simulink library "sm_excv_underc_lib"  (R2023b)
settings: Solver=VariableStepAuto  StartTime=0.0  StopTime=10.0  RelTol=1e-3
undefined symbols (not defined in the file): Excv, L1, L2, L3, L4, L5, L6, L7, L8, L9, P1, P2, P3, P4, P5, P6, P7, P8, P9, shoe_w, X, Y, Z
libraries: sm_tracked_vehicle_lib x70, sm_lib x54, nesl_utility x32, sm_excv_scene_lib x9, fl_lib x8, sm_excv_frame_lib x4
(part 1 of 5)
Description:
  | Copyright 2023 The MathWorks, Inc.
settings Model: Creator=smiller  LastModifiedBy=smiller

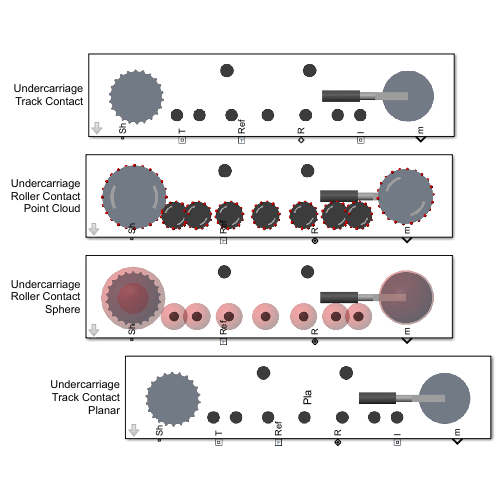
[thumbnail: Simulink's stored preview of the top-level diagram]
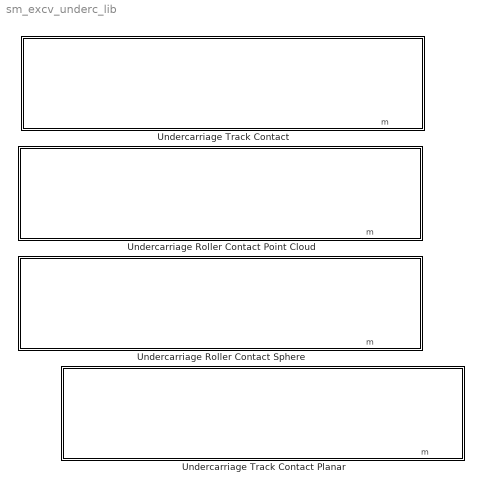
== system sm_excv_underc_lib ==
  Undercarriage Roller Contact Point Cloud : Subsystem  mask(Undercarriage with Roller Ground Contact (Point Cloud)){sprk_xc=Excv.Sprocket.sprocket_xc, sprk_len=Excv.Sprocket.sprk_width, sprk_rho=Excv.Sprocket.density, sprk_clr=Excv.Sprocket.clr, sprk_opc=Excv.Sprocket.opc, sprk_contact_geo_ptcld=Excv.Sprocket.ground_contact.ptcld.pts, sprk_contact_geo_rad=Excv.Sprocket.ground_contact.ptcld.rad, sprk_contact_geo_clr=Excv.Sprocket.ground_contact.ptcld.clr, sprk_contact_geo_opc=Excv.Sprocket.ground_contact.ptcld.opc, idler_rad=Excv.Idler.rad, idler_len=Excv.Idler.len, idler_rho=Excv.Idler.rho, idler_clr=Excv.Idler.clr, idler_opc=Excv.Idler.opc, idler_contact_geo_ptcld=Excv.Idler.ground_contact.ptcld.pts, idler_contact_geo_rad=Excv.Idler.ground_contact.ptcld.rad, idler_contact_geo_clr=Excv.Idler.ground_contact.ptcld.clr, idler_contact_geo_opc=Excv.Idler.ground_contact.ptcld.opc, roller_upper_rad=Excv.Roller.Upper.rad, roller_upper_len=Excv.Roller.Upper.len, roller_upper_rho=Excv.Roller.Upper.rho, roller_upper_clr=Excv.Roller.Upper.clr, roller_upper_opc=Excv.Roller.Upper.opc, roller_upper_contgeo_clr=[1.0 0.0 0.0], roller_upper_contgeo_opc=1, roller_lower_rad=Excv.Roller.Lower.rad, roller_lower_len=Excv.Roller.Lower.len, roller_lower_rho=Excv.Roller.Lower.rho, roller_lower_clr=Excv.Roller.Lower.clr, roller_lower_opc=Excv.Roller.Lower.opc, roller_lower_contgeo_ptcld=Excv.Roller.Lower.ground_contact.ptcld.pts, roller_lower_contgeo_rad=Excv.Roller.Lower.ground_contact.ptcld.rad, roller_lower_contgeo_clr=Excv.Roller.Lower.ground_contact.ptcld.clr, roller_lower_contgeo_opc=Excv.Roller.Lower.ground_contact.ptcld.opc, tensioner_cyl_len=Excv.Idler.Tensioner.cyl.len, tensioner_cyl_rad=Excv.Idler.Tensioner.cyl.rad, tensioner_cyl_rho=Excv.Idler.Tensioner.cyl.rho, tensioner_cyl_clr=Excv.Idler.Tensioner.cyl.clr, tensioner_cyl_opc=Excv.Idler.Tensioner.cyl.opc, tensioner_pist_len=Excv.Idler.Tensioner.piston.len, tensioner_pist_rad=Excv.Idler.Tensioner.piston.rad, tensioner_pist_rho=Excv.Idler.Tensioner.piston.rho, tensioner_pist_clr=Excv.Idler.Tensioner.piston.clr, tensioner_pist_opc=Excv.Idler.Tensioner.piston.opc, tensioner_br_length=Excv.Idler.Tensioner.bracket.len, tensioner_br_width=Excv.Idler.Tensioner.bracket.wid, tensioner_br_height=Excv.Idler.Tensioner.bracket.height, tensioner_br_thk=Excv.Idler.Tensioner.bracket.thk, tensioner_br_rho=Excv.Idler.Tensioner.bracket.rho, tensioner_br_clr=Excv.Idler.Tensioner.bracket.clr, tensioner_br_opc=Excv.Idler.Tensioner.bracket.opc, idler_max_ext=Excv.Idler.Tensioner.cyl.max_ext, sprk_rolling_rad=Excv.Sprocket.ground_contact.rolling_radius, idler_rolling_rad=Excv.Idler.ground_contact.rolling_radius, roller_lower_rolling_rad=Excv.Roller.Lower.ground_contact.rolling_radius, cyl_len=Excv.Shoe.w, lext=1e-3, roller_cyl_clr=Excv.Roller.Lower.clr, roller_cyl_opc=1, sprocket_cyl_clr=Excv.Sprocket.clr, sprocket_cyl_opc=1, idler_cyl_clr=Excv.Idler.clr, idler_cyl_opc=1, accMn=0.65, accMx=0.75, acc_clr=[0.8 0.8 0.8], acc_opc=1, roller_upper_x=Excv.Frame.Sprk2UpperX, roller_lower_x=Excv.Frame.Sprk2LowerX, idler_x=Excv.Frame.IdlerAssyX, roller_upper_y=Excv.Frame.Sprk2UpperY, plate_h=Excv.Chain.plate_h, sprk_pitch_rad=Excv.Sprocket.sprocket_rPitch, idler_lower_roller_offset_y=Excv.Frame.IdlerRollerVoffset, popup_sense_roller=Actuator Torque}
      mask prompts: sprk_xc "Extrusion Data [x y] (m)"; sprk_len "Length (m)"; sprk_rho "Density (kg/m^3)"; sprk_clr "Color [R G B] (0-1)"; sprk_opc "Opacity (0-1)"; sprk_contact_geo_ptcld "Point Cloud Data [x y z] (m)"; sprk_contact_geo_rad "Radius (m)"; sprk_contact_geo_clr "Color [R G B] (0-1)"; sprk_contact_geo_opc "Opacity (0-1)"; idler_rad "Idler Radius (m)"; idler_len "Length (m)"; idler_rho "Density (kg/m^3)"; idler_clr "Color [R G B] (0-1)"; idler_opc "Opacity (0-1)"; idler_contact_geo_ptcld "Point Cloud Data [x y z] (m)"; idler_contact_geo_rad "Point Radius (m)"; idler_contact_geo_clr "Color [R G B] (0-1)"; idler_contact_geo_opc "Opacity (0-1)"; roller_upper_rad "Radius (m)"; roller_upper_len "Length (m)"; roller_upper_rho "Density (kg/m^3)"; roller_upper_clr "Color [R G B] (0-1)"; roller_upper_opc "Opacity (0-1)"; roller_upper_contgeo_clr "Color [R G B] (0-1)"; roller_upper_contgeo_opc "Opacity (0-1)"; roller_lower_rad "Lower Roller Radius (m)"; roller_lower_len "Length (m)"; roller_lower_rho "Density (kg/m^3)"; roller_lower_clr "Color [R G B] (0-1)"; roller_lower_opc "Opacity (0-1)"; roller_lower_contgeo_ptcld "Point Cloud [x y z] (m)"; roller_lower_contgeo_rad "Point Radius (m)"; roller_lower_contgeo_clr "Color [R G B] (0-1)"; roller_lower_contgeo_opc "Opacity (0-1)"; tensioner_cyl_len "Length (m)"; tensioner_cyl_rad "Radius (m)"; tensioner_cyl_rho "Density (kg/m^3)"; tensioner_cyl_clr "Color [R G B] (0-1)"; tensioner_cyl_opc "Opacity (0-1)"; tensioner_pist_len "Length (m)"; tensioner_pist_rad "Radius (m)"; tensioner_pist_rho "Density (kg/m^3)"; tensioner_pist_clr "Color [R G B] (0-1)"; tensioner_pist_opc "Opacity (0.1)"; tensioner_br_length "Length (m)"; tensioner_br_width "Width (m)"; tensioner_br_height "Height (m)"; tensioner_br_thk "Thickness (m)"; tensioner_br_rho "Density (kg/m^3)"; tensioner_br_clr "Color [R G B] (0-1)"; tensioner_br_opc "Opacity (0.1)"; idler_max_ext "Max Extension in Track (m)"; sprk_rolling_rad "Sprocket Rolling Radius (m)"; idler_rolling_rad "Idler Rolling Radius (m)"; roller_lower_rolling_rad "Lower Roller Rolling Radius (m)"; cyl_len "Track Width (m)"; lext "Length Extensions (m)"; roller_cyl_clr "Cylinder Color [R G B] (0-1)"; roller_cyl_opc "Cylinder Opacity (0-1)"; sprocket_cyl_clr "Cylinder Color [R G B] (0-1)"; sprocket_cyl_opc "Cylinder Opacity (0-1)"; idler_cyl_clr "Cylinder Color [R G B] (0-1)"; idler_cyl_opc "Cylinder Opacity (0-1)"; accMn "Accent Min Radius (0-1)"; accMx "Accent Max Radius (0-1)"; acc_clr "Accent Color [R G B] (0-1)"; acc_opc "Accent Opacity (0-1)"; roller_upper_x "Upper Rollers (vector) (m)"; roller_lower_x "Lower Rollers (vector) (m)"; idler_x "Idler Wheel (m)"; roller_upper_y "Sprocket to Upper Rollers (m)"; plate_h "Chain Plate Height (m)"; sprk_pitch_rad "Sprocket Pitch Radius (m)"; idler_lower_roller_offset_y "Idler to Lower Roller Offset (lower edge) (m)"; popup_sense_roller "Roller"
      mask help: Models sprocket, rollers, and idler. Components have point cloud contact geometry to enable undercarriage to roll along uneven ground. The sprocket has a 1D rotational mechanical interface to the drivetrain.
      mask TypeOptions sprk_xc: Rollers/sprk_xc
      mask TypeOptions sprk_len: Rollers/sprk_len
      mask TypeOptions sprk_rho: Rollers/sprk_rho
      mask TypeOptions sprk_clr: Rollers/sprk_clr
      mask TypeOptions sprk_opc: Rollers/sprk_opc
      mask TypeOptions sprk_contact_geo_ptcld: Rollers/sprk_contact_geo_ptcld
      mask TypeOptions sprk_contact_geo_rad: Rollers/sprk_contact_geo_rad
      mask TypeOptions sprk_contact_geo_clr: Rollers/sprk_contact_geo_clr
      mask TypeOptions sprk_contact_geo_opc: Rollers/sprk_contact_geo_opc
      mask TypeOptions idler_rad: Frame/idler_rad | Rollers/idler_rad
      mask TypeOptions idler_len: Rollers/idler_len
      mask TypeOptions idler_rho: Rollers/idler_rho
      mask TypeOptions idler_clr: Rollers/idler_clr
      mask TypeOptions idler_opc: Rollers/idler_opc
      mask TypeOptions idler_contact_geo_ptcld: Rollers/idler_contact_geo_ptcld
      mask TypeOptions idler_contact_geo_rad: Rollers/idler_contact_geo_rad
      mask TypeOptions idler_contact_geo_clr: Rollers/idler_contact_geo_clr
      mask TypeOptions idler_contact_geo_opc: Rollers/idler_contact_geo_opc
      mask TypeOptions roller_upper_rad: Rollers/roller_upper_rad
      mask TypeOptions roller_upper_len: Rollers/roller_upper_len
      mask TypeOptions roller_upper_rho: Rollers/roller_upper_rho
      mask TypeOptions roller_upper_clr: Rollers/roller_upper_clr
      mask TypeOptions roller_upper_opc: Rollers/roller_upper_opc
      mask TypeOptions roller_upper_contgeo_clr: Rollers/roller_upper_contgeo_clr
      mask TypeOptions roller_upper_contgeo_opc: Rollers/roller_upper_contgeo_opc
      mask TypeOptions roller_lower_rad: Frame/roller_lower_rad | Rollers/roller_lower_rad
      mask TypeOptions roller_lower_len: Rollers/roller_lower_len
      mask TypeOptions roller_lower_rho: Rollers/roller_lower_rho
      mask TypeOptions roller_lower_clr: Rollers/roller_lower_clr
      mask TypeOptions roller_lower_opc: Rollers/roller_lower_opc
      mask TypeOptions roller_lower_contgeo_ptcld: Rollers/roller_lower_contgeo_ptcld
      mask TypeOptions roller_lower_contgeo_rad: Rollers/roller_lower_contgeo_rad
      mask TypeOptions roller_lower_contgeo_clr: Rollers/roller_lower_contgeo_clr
      mask TypeOptions roller_lower_contgeo_opc: Rollers/roller_lower_contgeo_opc
      mask TypeOptions tensioner_cyl_len: Rollers/tensioner_cyl_len
      mask TypeOptions tensioner_cyl_rad: Rollers/tensioner_cyl_rad
      mask TypeOptions tensioner_cyl_rho: Rollers/tensioner_cyl_rho
      mask TypeOptions tensioner_cyl_clr: Rollers/tensioner_cyl_clr
      mask TypeOptions tensioner_cyl_opc: Rollers/tensioner_cyl_opc
      mask TypeOptions tensioner_pist_len: Rollers/tensioner_pist_len
      mask TypeOptions tensioner_pist_rad: Rollers/tensioner_pist_rad
      mask TypeOptions tensioner_pist_rho: Rollers/tensioner_pist_rho
      mask TypeOptions tensioner_pist_clr: Rollers/tensioner_pist_clr
      mask TypeOptions tensioner_pist_opc: Rollers/tensioner_pist_opc
      mask TypeOptions tensioner_br_length: Rollers/tensioner_br_length
      mask TypeOptions tensioner_br_width: Rollers/tensioner_br_width
      mask TypeOptions tensioner_br_height: Rollers/tensioner_br_height
      mask TypeOptions tensioner_br_thk: Rollers/tensioner_br_thk
      mask TypeOptions tensioner_br_rho: Rollers/tensioner_br_rho
      mask TypeOptions tensioner_br_clr: Rollers/tensioner_br_clr
      mask TypeOptions tensioner_br_opc: Rollers/tensioner_br_opc
      mask TypeOptions idler_max_ext: Rollers/idler_max_ext
      mask TypeOptions sprk_rolling_rad: Rollers/sprk_rolling_rad
      mask TypeOptions idler_rolling_rad: Rollers/idler_rolling_rad
      mask TypeOptions roller_lower_rolling_rad: Rollers/roller_lower_rolling_rad
      mask TypeOptions cyl_len: Rollers/cyl_len
      mask TypeOptions lext: Rollers/lext
      mask TypeOptions roller_cyl_clr: Rollers/roller_cyl_clr
      mask TypeOptions roller_cyl_opc: Rollers/roller_cyl_opc
      mask TypeOptions sprocket_cyl_clr: Rollers/sprocket_cyl_clr
      mask TypeOptions sprocket_cyl_opc: Rollers/sprocket_cyl_opc
      mask TypeOptions idler_cyl_clr: Rollers/idler_cyl_clr
      mask TypeOptions idler_cyl_opc: Rollers/idler_cyl_opc
      mask TypeOptions accMn: Rollers/accMn
      mask TypeOptions accMx: Rollers/accMx
      mask TypeOptions acc_clr: Rollers/acc_clr
      mask TypeOptions acc_opc: Rollers/acc_opc
      mask TypeOptions roller_upper_x: Frame/roller_upper_x
      mask TypeOptions roller_lower_x: Frame/roller_lower_x
      mask TypeOptions idler_x: Frame/idler_x
      mask TypeOptions roller_upper_y: Frame/roller_upper_y
      mask TypeOptions plate_h: Frame/plate_h
      mask TypeOptions sprk_pitch_rad: Frame/sprk_pitch_rad
      mask TypeOptions idler_lower_roller_offset_y: Frame/idler_lower_roller_offset_y
      mask TypeOptions popup_sense_roller: Rollers/popup_sense_roller
      mask DialogControl cont_sprocket Prompt: Sprocket
      mask DialogControl cont_sprocket_solid Prompt: Solid
      mask DialogControl cont_sprocket_contact_geo Prompt: Contact Geometry
      mask DialogControl cont_idler Prompt: Idler
      mask DialogControl cont_idler_solid Prompt: Solid
      mask DialogControl cont_idler_contact_geo Prompt: Contact Geometry
      mask DialogControl cont_rollers Prompt: Rollers
      mask DialogControl cont_roller_upper Prompt: Upper
      mask DialogControl cont_roller_upper_contact_geo Prompt: Contact Geometry
      mask DialogControl cont_rollers_lower Prompt: Lower
      mask DialogControl cont_rollers_lower_contact_geo Prompt: Contact Geometry
      mask DialogControl cont_tensioner Prompt: Tensioner
      mask DialogControl cont_tensioner_cyl Prompt: Cylinder
      mask DialogControl cont_tensioner_pist Prompt: Piston
      mask DialogControl cont_tensioner_brkt Prompt: Bracket
      mask DialogControl cont_tensioner_assembly Prompt: Assembly
      mask DialogControl cont_rolling Prompt: Rolling
      mask DialogControl cont_rolling_constr_len Prompt: Constraints and Length
      mask DialogControl cont_rollvis_roller Prompt: Roller Visual: Roller
      mask DialogControl cont_rollvis_sprk Prompt: Roller Visual: Sprocket
      mask DialogControl cont_rollvis_idler Prompt: Roller Visual: Idler
      mask DialogControl cont_accvis Prompt: Accent Visual
      mask DialogControl cont_frame Prompt: Frame
      mask DialogControl cont_offset_x Prompt: Longitudinal Offsets from Sprocket
      mask DialogControl cont_offset_y Prompt: Vertical Offsets
      mask DialogControl cont_sensing Prompt: Sensing
      mask Display: image('sm_excv_track_rollersptcld_IMAGE.png');
  Undercarriage Roller Contact Sphere : Subsystem  mask(Undercarriage with Roller Ground Contact (Spheres)){sprk_xc=Excv.Sprocket.sprocket_xc, sprk_len=Excv.Sprocket.sprk_width, sprk_rho=Excv.Sprocket.density, sprk_clr=Excv.Sprocket.clr, sprk_opc=Excv.Sprocket.opc, sprk_contact_geo_clr=Excv.Sprocket.ground_contact.sphere.clr, sprk_contact_geo_opc=Excv.Sprocket.ground_contact.sphere.opc, idler_rad=Excv.Idler.rad, idler_len=Excv.Idler.len, idler_rho=Excv.Idler.rho, idler_clr=Excv.Idler.clr, idler_opc=Excv.Idler.opc, idler_contact_geo_clr=Excv.Idler.ground_contact.sphere.clr, idler_contact_geo_opc=Excv.Idler.ground_contact.sphere.opc, roller_upper_rad=Excv.Roller.Upper.rad, roller_upper_len=Excv.Roller.Upper.len, roller_upper_rho=Excv.Roller.Upper.rho, roller_upper_clr=Excv.Roller.Upper.clr, roller_upper_opc=Excv.Roller.Upper.opc, roller_upper_contgeo_clr=[1.0 0.0 0.0], roller_upper_contgeo_opc=1, roller_lower_rad=Excv.Roller.Lower.rad, roller_lower_len=Excv.Roller.Lower.len, roller_lower_rho=Excv.Roller.Lower.rho, roller_lower_clr=Excv.Roller.Lower.clr, roller_lower_opc=Excv.Roller.Lower.opc, roller_lower_contgeo_clr=Excv.Roller.Lower.ground_contact.sphere.clr, roller_lower_contgeo_opc=Excv.Roller.Lower.ground_contact.sphere.opc, tensioner_cyl_len=Excv.Idler.Tensioner.cyl.len, tensioner_cyl_rad=Excv.Idler.Tensioner.cyl.rad, tensioner_cyl_rho=Excv.Idler.Tensioner.cyl.rho, tensioner_cyl_clr=Excv.Idler.Tensioner.cyl.clr, tensioner_cyl_opc=Excv.Idler.Tensioner.cyl.opc, tensioner_pist_len=Excv.Idler.Tensioner.piston.len, tensioner_pist_rad=Excv.Idler.Tensioner.piston.rad, tensioner_pist_rho=Excv.Idler.Tensioner.piston.rho, tensioner_pist_clr=Excv.Idler.Tensioner.piston.clr, tensioner_pist_opc=Excv.Idler.Tensioner.piston.opc, tensioner_br_length=Excv.Idler.Tensioner.bracket.len, tensioner_br_width=Excv.Idler.Tensioner.bracket.wid, tensioner_br_height=Excv.Idler.Tensioner.bracket.height, tensioner_br_thk=Excv.Idler.Tensioner.bracket.thk, tensioner_br_rho=Excv.Idler.Tensioner.bracket.rho, tensioner_br_clr=Excv.Idler.Tensioner.bracket.clr, tensioner_br_opc=Excv.Idler.Tensioner.bracket.opc, idler_max_ext=Excv.Idler.Tensioner.cyl.max_ext, sprk_rolling_rad=Excv.Sprocket.ground_contact.rolling_radius, idler_rolling_rad=Excv.Idler.ground_contact.rolling_radius, roller_lower_rolling_rad=Excv.Roller.Lower.ground_contact.rolling_radius, shoe_w=shoe_w, roller_upper_x=Excv.Frame.Sprk2UpperX, roller_lower_x=Excv.Frame.Sprk2LowerX, idler_x=Excv.Frame.IdlerAssyX, roller_upper_y=Excv.Frame.Sprk2UpperY, plate_h=Excv.Chain.plate_h, sprk_pitch_rad=Excv.Sprocket.sprocket_rPitch, idler_lower_roller_offset_y=Excv.Frame.IdlerRollerVoffset, popup_sense_roller=Actuator Torque}
      mask prompts: sprk_xc "Extrusion Data [x y] (m)"; sprk_len "Length (m)"; sprk_rho "Density (kg/m^3)"; sprk_clr "Color [R G B] (0-1)"; sprk_opc "Opacity (0-1)"; sprk_contact_geo_clr "Color [R G B] (0-1)"; sprk_contact_geo_opc "Opacity (0-1)"; idler_rad "Idler Radius (m)"; idler_len "Length (m)"; idler_rho "Density (kg/m^3)"; idler_clr "Color [R G B] (0-1)"; idler_opc "Opacity (0-1)"; idler_contact_geo_clr "Color [R G B] (0-1)"; idler_contact_geo_opc "Opacity (0-1)"; roller_upper_rad "Radius (m)"; roller_upper_len "Length (m)"; roller_upper_rho "Density (kg/m^3)"; roller_upper_clr "Color [R G B] (0-1)"; roller_upper_opc "Opacity (0-1)"; roller_upper_contgeo_clr "Color [R G B] (0-1)"; roller_upper_contgeo_opc "Opacity (0-1)"; roller_lower_rad "Lower Roller Radius (m)"; roller_lower_len "Length (m)"; roller_lower_rho "Density (kg/m^3)"; roller_lower_clr "Color [R G B] (0-1)"; roller_lower_opc "Opacity (0-1)"; roller_lower_contgeo_clr "Color [R G B] (0-1)"; roller_lower_contgeo_opc "Opacity (0-1)"; tensioner_cyl_len "Length (m)"; tensioner_cyl_rad "Radius (m)"; tensioner_cyl_rho "Density (kg/m^3)"; tensioner_cyl_clr "Color [R G B] (0-1)"; tensioner_cyl_opc "Opacity (0-1)"; tensioner_pist_len "Length (m)"; tensioner_pist_rad "Radius (m)"; tensioner_pist_rho "Density (kg/m^3)"; tensioner_pist_clr "Color [R G B] (0-1)"; tensioner_pist_opc "Opacity (0.1)"; tensioner_br_length "Length (m)"; tensioner_br_width "Width (m)"; tensioner_br_height "Height (m)"; tensioner_br_thk "Thickness (m)"; tensioner_br_rho "Density (kg/m^3)"; tensioner_br_clr "Color [R G B] (0-1)"; tensioner_br_opc "Opacity (0.1)"; idler_max_ext "Max Extension in Track (m)"; sprk_rolling_rad "Sprocket Rolling Radius (m)"; idler_rolling_rad "Idler Rolling Radius (m)"; roller_lower_rolling_rad "Lower Roller Rolling Radius (m)"; shoe_w "Shoe Width (m)"; roller_upper_x "Upper Rollers (vector) (m)"; roller_lower_x "Lower Rollers (vector) (m)"; idler_x "Idler Wheel (m)"; roller_upper_y "Sprocket to Upper Rollers (m)"; plate_h "Chain Plate Height (m)"; sprk_pitch_rad "Sprocket Pitch Radius (m)"; idler_lower_roller_offset_y "Idler to Lower Roller Offset (lower edge) (m)"; popup_sense_roller "Roller"
      mask help: Models sprocket, rollers, and idler. Components have sphere contact geometry to enable undercarriage to roll along uneven ground. The sprocket has a 1D rotational mechanical interface to the drivetrain.
      mask TypeOptions sprk_xc: Rollers/sprk_xc
      mask TypeOptions sprk_len: Rollers/sprk_len
      mask TypeOptions sprk_rho: Rollers/sprk_rho
      mask TypeOptions sprk_clr: Rollers/sprk_clr
      mask TypeOptions sprk_opc: Rollers/sprk_opc
      mask TypeOptions sprk_contact_geo_clr: Rollers/sprk_contact_geo_clr
      mask TypeOptions sprk_contact_geo_opc: Rollers/sprk_contact_geo_opc
      mask TypeOptions idler_rad: Frame/idler_rad | Rollers/idler_rad
      mask TypeOptions idler_len: Rollers/idler_len
      mask TypeOptions idler_rho: Rollers/idler_rho
      mask TypeOptions idler_clr: Rollers/idler_clr
      mask TypeOptions idler_opc: Rollers/idler_opc
      mask TypeOptions idler_contact_geo_clr: Rollers/idler_contact_geo_clr
      mask TypeOptions idler_contact_geo_opc: Rollers/idler_contact_geo_opc
      mask TypeOptions roller_upper_rad: Rollers/roller_upper_rad
      mask TypeOptions roller_upper_len: Rollers/roller_upper_len
      mask TypeOptions roller_upper_rho: Rollers/roller_upper_rho
      mask TypeOptions roller_upper_clr: Rollers/roller_upper_clr
      mask TypeOptions roller_upper_opc: Rollers/roller_upper_opc
      mask TypeOptions roller_upper_contgeo_clr: Rollers/roller_upper_contgeo_clr
      mask TypeOptions roller_upper_contgeo_opc: Rollers/roller_upper_contgeo_opc
      mask TypeOptions roller_lower_rad: Frame/roller_lower_rad | Rollers/roller_lower_rad
      mask TypeOptions roller_lower_len: Rollers/roller_lower_len
      mask TypeOptions roller_lower_rho: Rollers/roller_lower_rho
      mask TypeOptions roller_lower_clr: Rollers/roller_lower_clr
      mask TypeOptions roller_lower_opc: Rollers/roller_lower_opc
      mask TypeOptions roller_lower_contgeo_clr: Rollers/roller_lower_contgeo_clr
      mask TypeOptions roller_lower_contgeo_opc: Rollers/roller_lower_contgeo_opc
      mask TypeOptions tensioner_cyl_len: Rollers/tensioner_cyl_len
      mask TypeOptions tensioner_cyl_rad: Rollers/tensioner_cyl_rad
      mask TypeOptions tensioner_cyl_rho: Rollers/tensioner_cyl_rho
      mask TypeOptions tensioner_cyl_clr: Rollers/tensioner_cyl_clr
      mask TypeOptions tensioner_cyl_opc: Rollers/tensioner_cyl_opc
      mask TypeOptions tensioner_pist_len: Rollers/tensioner_pist_len
      mask TypeOptions tensioner_pist_rad: Rollers/tensioner_pist_rad
      mask TypeOptions tensioner_pist_rho: Rollers/tensioner_pist_rho
      mask TypeOptions tensioner_pist_clr: Rollers/tensioner_pist_clr
      mask TypeOptions tensioner_pist_opc: Rollers/tensioner_pist_opc
      mask TypeOptions tensioner_br_length: Rollers/tensioner_br_length
      mask TypeOptions tensioner_br_width: Rollers/tensioner_br_width
      mask TypeOptions tensioner_br_height: Rollers/tensioner_br_height
      mask TypeOptions tensioner_br_thk: Rollers/tensioner_br_thk
      mask TypeOptions tensioner_br_rho: Rollers/tensioner_br_rho
      mask TypeOptions tensioner_br_clr: Rollers/tensioner_br_clr
      mask TypeOptions tensioner_br_opc: Rollers/tensioner_br_opc
      mask TypeOptions idler_max_ext: Rollers/idler_max_ext
      mask TypeOptions sprk_rolling_rad: Rollers/sprk_rolling_rad
      mask TypeOptions idler_rolling_rad: Rollers/idler_rolling_rad
      mask TypeOptions roller_lower_rolling_rad: Rollers/roller_lower_rolling_rad
      mask TypeOptions shoe_w: Rollers/shoe_w
      mask TypeOptions roller_upper_x: Frame/roller_upper_x
      mask TypeOptions roller_lower_x: Frame/roller_lower_x
      mask TypeOptions idler_x: Frame/idler_x
      mask TypeOptions roller_upper_y: Frame/roller_upper_y
      mask TypeOptions plate_h: Frame/plate_h
      mask TypeOptions sprk_pitch_rad: Frame/sprk_pitch_rad
      mask TypeOptions idler_lower_roller_offset_y: Frame/idler_lower_roller_offset_y
      mask TypeOptions popup_sense_roller: Rollers/popup_sense_roller
      mask DialogControl cont_sprocket Prompt: Sprocket
      mask DialogControl cont_sprocket_solid Prompt: Solid
      mask DialogControl cont_sprocket_contact_geo Prompt: Contact Geometry
      mask DialogControl cont_idler Prompt: Idler
      mask DialogControl cont_idler_solid Prompt: Solid
      mask DialogControl cont_idler_contact_geo Prompt: Contact Geometry
      mask DialogControl cont_rollers Prompt: Rollers
      mask DialogControl cont_roller_upper Prompt: Upper
      mask DialogControl cont_roller_upper_contact_geo Prompt: Contact Geometry
      mask DialogControl cont_rollers_lower Prompt: Lower
      mask DialogControl cont_rollers_lower_contact_geo Prompt: Contact Geometry
      mask DialogControl cont_tensioner Prompt: Tensioner
      mask DialogControl cont_tensioner_cyl Prompt: Cylinder
      mask DialogControl cont_tensioner_pist Prompt: Piston
      mask DialogControl cont_tensioner_brkt Prompt: Bracket
      mask DialogControl cont_tensioner_assembly Prompt: Assembly
      mask DialogControl cont_rolling Prompt: Rolling
      mask DialogControl cont_const_len Prompt: Constraints and Length
      mask DialogControl cont_frame Prompt: Frame
      mask DialogControl cont_offset_x Prompt: Longitudinal Offsets from Sprocket
      mask DialogControl cont_offset_y Prompt: Vertical Offsets
      mask DialogControl cont_sensing Prompt: Sensing
      mask Display: image('sm_excv_track_rollerssphere_IMAGE.png');
  Undercarriage Track Contact : Subsystem  mask(Undercarriage for Integration with Track Model){sprk_xc=Excv.Sprocket.sprocket_xc, sprk_len=Excv.Sprocket.sprk_width, sprk_rho=Excv.Sprocket.density, sprk_clr=Excv.Sprocket.clr, sprk_opc=Excv.Sprocket.opc, sprk_contact_geo_ptcld=Excv.Sprocket.teeth_contact.ptcld.pts, sprk_contact_geo_rad=Excv.Sprocket.teeth_contact.ptcld.rad, sprk_contact_geo_clr=Excv.Sprocket.teeth_contact.ptcld.clr, sprk_contact_geo_opc=Excv.Sprocket.teeth_contact.ptcld.opc, idler_rad=Excv.Idler.rad, idler_len=Excv.Idler.len, idler_rho=Excv.Idler.rho, idler_clr=Excv.Idler.clr, idler_opc=Excv.Idler.opc, idler_contgeo_clr=Excv.Idler.chain_contact.clr, idler_contgeo_opc=Excv.Idler.chain_contact.opc, roller_upper_rad=Excv.Roller.Upper.rad, roller_upper_len=Excv.Roller.Upper.len, roller_upper_rho=Excv.Roller.Upper.rho, roller_upper_clr=Excv.Roller.Upper.clr, roller_upper_opc=Excv.Roller.Upper.opc, roller_upper_contgeo_clr=[1.0 0.0 0.0], roller_upper_contgeo_opc=1, roller_lower_rad=Excv.Roller.Lower.rad, roller_lower_len=Excv.Roller.Lower.len, roller_lower_rho=Excv.Roller.Lower.rho, roller_lower_clr=Excv.Roller.Lower.clr, roller_lower_opc=Excv.Roller.Lower.opc, roller_lower_contgeo_clr=[1.0 0.0 0.0], roller_lower_contgeo_opc=1, tensioner_cyl_len=Excv.Idler.Tensioner.cyl.len, tensioner_cyl_rad=Excv.Idler.Tensioner.cyl.rad, tensioner_cyl_rho=Excv.Idler.Tensioner.cyl.rho, tensioner_cyl_clr=Excv.Idler.Tensioner.cyl.clr, tensioner_cyl_opc=Excv.Idler.Tensioner.cyl.opc, tensioner_pist_len=Excv.Idler.Tensioner.piston.len, tensioner_pist_rad=Excv.Idler.Tensioner.piston.rad, tensioner_pist_rho=Excv.Idler.Tensioner.piston.rho, tensioner_pist_clr=Excv.Idler.Tensioner.piston.clr, tensioner_pist_opc=Excv.Idler.Tensioner.piston.opc, tensioner_br_length=Excv.Idler.Tensioner.bracket.len, tensioner_br_width=Excv.Idler.Tensioner.bracket.wid, tensioner_br_height=Excv.Idler.Tensioner.bracket.height, tensioner_br_thk=Excv.Idler.Tensioner.bracket.thk, tensioner_br_rho=Excv.Idler.Tensioner.bracket.rho, tensioner_br_clr=Excv.Idler.Tensioner.bracket.clr, tensioner_br_opc=Excv.Idler.Tensioner.bracket.opc, tensioner_eqpos=Excv.Idler.Tensioner.xeq, tensioner_x0=Excv.Idler.Tensioner.x0, tensioner_k=Excv.Idler.Tensioner.K, tensioner_b=Excv.Idler.Tensioner.B, roller_upper_x=Excv.Frame.Sprk2UpperX, roller_lower_x=Excv.Frame.Sprk2LowerX, idler_x=Excv.Frame.IdlerAssyX, roller_upper_y=Excv.Frame.Sprk2UpperY, plate_h=Excv.Chain.plate_h, sprk_pitch_rad=Excv.Sprocket.sprocket_rPitch, idler_lower_roller_offset_y=Excv.Frame.IdlerRollerVoffset, popup_sense_roller=Actuator Torque}
      mask prompts: sprk_xc "Extrusion Data [x y] (m)"; sprk_len "Length (m)"; sprk_rho "Density (kg/m^3)"; sprk_clr "Color [R G B] (0-1)"; sprk_opc "Opacity (0-1)"; sprk_contact_geo_ptcld "Point Cloud Data [x y z] (m)"; sprk_contact_geo_rad "Radius (m)"; sprk_contact_geo_clr "Color [R G B] (0-1)"; sprk_contact_geo_opc "Opacity (0-1)"; idler_rad "Idler Radius (m)"; idler_len "Length (m)"; idler_rho "Density (kg/m^3)"; idler_clr "Color [R G B] (0-1)"; idler_opc "Opacity (0-1)"; idler_contgeo_clr "Color [R G B] (0-1)"; idler_contgeo_opc "Opacity (0-1)"; roller_upper_rad "Radius (m)"; roller_upper_len "Length (m)"; roller_upper_rho "Density (kg/m^3)"; roller_upper_clr "Color [R G B] (0-1)"; roller_upper_opc "Opacity (0-1)"; roller_upper_contgeo_clr "Color [R G B] (0-1)"; roller_upper_contgeo_opc "Opacity (0-1)"; roller_lower_rad "Lower Roller Radius (m)"; roller_lower_len "Length (m)"; roller_lower_rho "Density (kg/m^3)"; roller_lower_clr "Color [R G B] (0-1)"; roller_lower_opc "Opacity (0-1)"; roller_lower_contgeo_clr "Color [R G B] (0-1)"; roller_lower_contgeo_opc "Opacity (0-1)"; tensioner_cyl_len "Length (m)"; tensioner_cyl_rad "Radius (m)"; tensioner_cyl_rho "Density (kg/m^3)"; tensioner_cyl_clr "Color [R G B] (0-1)"; tensioner_cyl_opc "Opacity (0-1)"; tensioner_pist_len "Length (m)"; tensioner_pist_rad "Radius (m)"; tensioner_pist_rho "Density (kg/m^3)"; tensioner_pist_clr "Color [R G B] (0-1)"; tensioner_pist_opc "Opacity (0.1)"; tensioner_br_length "Length (m)"; tensioner_br_width "Width (m)"; tensioner_br_height "Height (m)"; tensioner_br_thk "Thickness (m)"; tensioner_br_rho "Density (kg/m^3)"; tensioner_br_clr "Color [R G B] (0-1)"; tensioner_br_opc "Opacity (0.1)"; tensioner_eqpos "Equilibrium Position (m)"; tensioner_x0 "Assembly Position (m)"; tensioner_k "Stiffness Coefficient (N/m)"; tensioner_b "Damping Coefficient (N/(m/s))"; roller_upper_x "Upper Rollers (vector) (m)"; roller_lower_x "Lower Rollers (vector) (m)"; idler_x "Idler Wheel (m)"; roller_upper_y "Sprocket to Upper Rollers (m)"; plate_h "Chain Plate Height (m)"; sprk_pitch_rad "Sprocket Pitch Radius (m)"; idler_lower_roller_offset_y "Idler to Lower Roller Offset (lower edge) (m)"; popup_sense_roller "Roller"
      mask help: Models sprocket, rollers, and idler with tensioner. Components have contact geometry for integration with a segmented track model. The sprocket has a 1D rotational mechanical interface to the drivetrain.
      mask TypeOptions sprk_xc: Rollers/sprk_xc
      mask TypeOptions sprk_len: Rollers/sprk_len
      mask TypeOptions sprk_rho: Rollers/sprk_rho
      mask TypeOptions sprk_clr: Rollers/sprk_clr
      mask TypeOptions sprk_opc: Rollers/sprk_opc
      mask TypeOptions sprk_contact_geo_ptcld: Rollers/sprk_contact_geo_ptcld
      mask TypeOptions sprk_contact_geo_rad: Rollers/sprk_contact_geo_rad
      mask TypeOptions sprk_contact_geo_clr: Rollers/sprk_contact_geo_clr
      mask TypeOptions sprk_contact_geo_opc: Rollers/sprk_contact_geo_opc
      mask TypeOptions idler_rad: Frame/idler_rad | Rollers/idler_rad
      mask TypeOptions idler_len: Rollers/idler_len
      mask TypeOptions idler_rho: Rollers/idler_rho
      mask TypeOptions idler_clr: Rollers/idler_clr
      mask TypeOptions idler_opc: Rollers/idler_opc
      mask TypeOptions idler_contgeo_clr: Rollers/idler_contgeo_clr
      mask TypeOptions idler_contgeo_opc: Rollers/idler_contgeo_opc
      mask TypeOptions roller_upper_rad: Rollers/roller_upper_rad
      mask TypeOptions roller_upper_len: Rollers/roller_upper_len
      mask TypeOptions roller_upper_rho: Rollers/roller_upper_rho
      mask TypeOptions roller_upper_clr: Rollers/roller_upper_clr
      mask TypeOptions roller_upper_opc: Rollers/roller_upper_opc
      mask TypeOptions roller_upper_contgeo_clr: Rollers/roller_upper_contgeo_clr
      mask TypeOptions roller_upper_contgeo_opc: Rollers/roller_upper_contgeo_opc
      mask TypeOptions roller_lower_rad: Frame/roller_lower_rad | Rollers/roller_lower_rad
      mask TypeOptions roller_lower_len: Rollers/roller_lower_len
      mask TypeOptions roller_lower_rho: Rollers/roller_lower_rho
      mask TypeOptions roller_lower_clr: Rollers/roller_lower_clr
      mask TypeOptions roller_lower_opc: Rollers/roller_lower_opc
      mask TypeOptions roller_lower_contgeo_clr: Rollers/roller_lower_contgeo_clr
      mask TypeOptions roller_lower_contgeo_opc: Rollers/roller_lower_contgeo_opc
      mask TypeOptions tensioner_cyl_len: Rollers/tensioner_cyl_len
      mask TypeOptions tensioner_cyl_rad: Rollers/tensioner_cyl_rad
      mask TypeOptions tensioner_cyl_rho: Rollers/tensioner_cyl_rho
      mask TypeOptions tensioner_cyl_clr: Rollers/tensioner_cyl_clr
      mask TypeOptions tensioner_cyl_opc: Rollers/tensioner_cyl_opc
      mask TypeOptions tensioner_pist_len: Rollers/tensioner_pist_len
      mask TypeOptions tensioner_pist_rad: Rollers/tensioner_pist_rad
      mask TypeOptions tensioner_pist_rho: Rollers/tensioner_pist_rho
      mask TypeOptions tensioner_pist_clr: Rollers/tensioner_pist_clr
      mask TypeOptions tensioner_pist_opc: Rollers/tensioner_pist_opc
      mask TypeOptions tensioner_br_length: Rollers/tensioner_br_length
      mask TypeOptions tensioner_br_width: Rollers/tensioner_br_width
      mask TypeOptions tensioner_br_height: Rollers/tensioner_br_height
      mask TypeOptions tensioner_br_thk: Rollers/tensioner_br_thk
      mask TypeOptions tensioner_br_rho: Rollers/tensioner_br_rho
      mask TypeOptions tensioner_br_clr: Rollers/tensioner_br_clr
      mask TypeOptions tensioner_br_opc: Rollers/tensioner_br_opc
      mask TypeOptions tensioner_eqpos: Rollers/tensioner_eqpos
      mask TypeOptions tensioner_x0: Rollers/tensioner_x0
      mask TypeOptions tensioner_k: Rollers/tensioner_k
      mask TypeOptions tensioner_b: Rollers/tensioner_b
      mask TypeOptions roller_upper_x: Frame/roller_upper_x
      mask TypeOptions roller_lower_x: Frame/roller_lower_x
      mask TypeOptions idler_x: Frame/idler_x
      mask TypeOptions roller_upper_y: Frame/roller_upper_y
      mask TypeOptions plate_h: Frame/plate_h
      mask TypeOptions sprk_pitch_rad: Frame/sprk_pitch_rad
      mask TypeOptions idler_lower_roller_offset_y: Frame/idler_lower_roller_offset_y
      mask TypeOptions popup_sense_roller: Rollers/popup_sense_roller
      mask DialogControl cont_sprocket Prompt: Sprocket
      mask DialogControl cont_sprocket_solid Prompt: Solid
      mask DialogControl cont_sprocket_contact_geo Prompt: Contact Geometry
      mask DialogControl cont_idler Prompt: Idler
      mask DialogControl cont_idler_solid Prompt: Solid
      mask DialogControl cont_idler_contact_geo Prompt: Contact Geometry
      mask DialogControl cont_rollers Prompt: Rollers
      mask DialogControl cont_roller_upper Prompt: Upper
      mask DialogControl cont_roller_upper_contact_geo Prompt: Contact Geometry
      mask DialogControl cont_rollers_lower Prompt: Lower
      mask DialogControl cont_rollers_lower_contact_geo Prompt: Contact Geometry
      mask DialogControl cont_tensioner Prompt: Tensioner
      mask DialogControl cont_tensioner_cyl Prompt: Cylinder
      mask DialogControl cont_tensioner_pist Prompt: Piston
      mask DialogControl cont_tensioner_brkt Prompt: Bracket
      mask DialogControl cont_tensioner_assembly Prompt: Assembly
      mask DialogControl cont_frame Prompt: Frame
      mask DialogControl cont_offset_x Prompt: Longitudinal Offsets from Sprocket
      mask DialogControl cont_offset_y Prompt: Vertical Offsets
      mask DialogControl cont_sensing Prompt: Sensing
      mask Display: image('sm_excv_track_rollers_IMAGE.png');
  Undercarriage Track Contact Planar : Subsystem  mask(Undercarriage for Integration with Track Model){sprk_xc=Excv.Sprocket.sprocket_xc, sprk_len=Excv.Sprocket.sprk_width, sprk_rho=Excv.Sprocket.density, sprk_clr=Excv.Sprocket.clr, sprk_opc=Excv.Sprocket.opc, sprk_contact_geo_ptcld=Excv.Sprocket.teeth_contact.ptcld.pts, sprk_contact_geo_rad=Excv.Sprocket.teeth_contact.ptcld.rad, sprk_contact_geo_clr=Excv.Sprocket.teeth_contact.ptcld.clr, sprk_contact_geo_opc=Excv.Sprocket.teeth_contact.ptcld.opc, idler_rad=Excv.Idler.rad, idler_len=Excv.Idler.len, idler_rho=Excv.Idler.rho, idler_clr=Excv.Idler.clr, idler_opc=Excv.Idler.opc, idler_contgeo_clr=Excv.Idler.chain_contact.clr, idler_contgeo_opc=Excv.Idler.chain_contact.opc, roller_upper_rad=Excv.Roller.Upper.rad, roller_upper_len=Excv.Roller.Upper.len, roller_upper_rho=Excv.Roller.Upper.rho, roller_upper_clr=Excv.Roller.Upper.clr, roller_upper_opc=Excv.Roller.Upper.opc, roller_upper_contgeo_clr=[1.0 0.0 0.0], roller_upper_contgeo_opc=1, roller_lower_rad=Excv.Roller.Lower.rad, roller_lower_len=Excv.Roller.Lower.len, roller_lower_rho=Excv.Roller.Lower.rho, roller_lower_clr=Excv.Roller.Lower.clr, roller_lower_opc=Excv.Roller.Lower.opc, roller_lower_contgeo_clr=[1.0 0.0 0.0], roller_lower_contgeo_opc=1, tensioner_cyl_len=Excv.Idler.Tensioner.cyl.len, tensioner_cyl_rad=Excv.Idler.Tensioner.cyl.rad, tensioner_cyl_rho=Excv.Idler.Tensioner.cyl.rho, tensioner_cyl_clr=Excv.Idler.Tensioner.cyl.clr, tensioner_cyl_opc=Excv.Idler.Tensioner.cyl.opc, tensioner_pist_len=Excv.Idler.Tensioner.piston.len, tensioner_pist_rad=Excv.Idler.Tensioner.piston.rad, tensioner_pist_rho=Excv.Idler.Tensioner.piston.rho, tensioner_pist_clr=Excv.Idler.Tensioner.piston.clr, tensioner_pist_opc=Excv.Idler.Tensioner.piston.opc, tensioner_br_length=Excv.Idler.Tensioner.bracket.len, tensioner_br_width=Excv.Idler.Tensioner.bracket.wid, tensioner_br_height=Excv.Idler.Tensioner.bracket.height, tensioner_br_thk=Excv.Idler.Tensioner.bracket.thk, tensioner_br_rho=Excv.Idler.Tensioner.bracket.rho, tensioner_br_clr=Excv.Idler.Tensioner.bracket.clr, tensioner_br_opc=Excv.Idler.Tensioner.bracket.opc, tensioner_eqpos=Excv.Idler.Tensioner.xeq, tensioner_x0=Excv.Idler.Tensioner.x0, tensioner_k=Excv.Idler.Tensioner.K, tensioner_b=Excv.Idler.Tensioner.B, roller_upper_x=Excv.Frame.Sprk2UpperX, roller_lower_x=Excv.Frame.Sprk2LowerX, idler_x=Excv.Frame.IdlerAssyX, roller_upper_y=Excv.Frame.Sprk2UpperY, plate_h=Excv.Chain.plate_h, sprk_pitch_rad=Excv.Sprocket.sprocket_rPitch, idler_lower_roller_offset_y=Excv.Frame.IdlerRollerVoffset, popup_sense_roller=Actuator Torque}
      mask prompts: sprk_xc "Extrusion Data [x y] (m)"; sprk_len "Length (m)"; sprk_rho "Density (kg/m^3)"; sprk_clr "Color [R G B] (0-1)"; sprk_opc "Opacity (0-1)"; sprk_contact_geo_ptcld "Point Cloud Data [x y z] (m)"; sprk_contact_geo_rad "Radius (m)"; sprk_contact_geo_clr "Color [R G B] (0-1)"; sprk_contact_geo_opc "Opacity (0-1)"; idler_rad "Idler Radius (m)"; idler_len "Length (m)"; idler_rho "Density (kg/m^3)"; idler_clr "Color [R G B] (0-1)"; idler_opc "Opacity (0-1)"; idler_contgeo_clr "Color [R G B] (0-1)"; idler_contgeo_opc "Opacity (0-1)"; roller_upper_rad "Radius (m)"; roller_upper_len "Length (m)"; roller_upper_rho "Density (kg/m^3)"; roller_upper_clr "Color [R G B] (0-1)"; roller_upper_opc "Opacity (0-1)"; roller_upper_contgeo_clr "Color [R G B] (0-1)"; roller_upper_contgeo_opc "Opacity (0-1)"; roller_lower_rad "Lower Roller Radius (m)"; roller_lower_len "Length (m)"; roller_lower_rho "Density (kg/m^3)"; roller_lower_clr "Color [R G B] (0-1)"; roller_lower_opc "Opacity (0-1)"; roller_lower_contgeo_clr "Color [R G B] (0-1)"; roller_lower_contgeo_opc "Opacity (0-1)"; tensioner_cyl_len "Length (m)"; tensioner_cyl_rad "Radius (m)"; tensioner_cyl_rho "Density (kg/m^3)"; tensioner_cyl_clr "Color [R G B] (0-1)"; tensioner_cyl_opc "Opacity (0-1)"; tensioner_pist_len "Length (m)"; tensioner_pist_rad "Radius (m)"; tensioner_pist_rho "Density (kg/m^3)"; tensioner_pist_clr "Color [R G B] (0-1)"; tensioner_pist_opc "Opacity (0.1)"; tensioner_br_length "Length (m)"; tensioner_br_width "Width (m)"; tensioner_br_height "Height (m)"; tensioner_br_thk "Thickness (m)"; tensioner_br_rho "Density (kg/m^3)"; tensioner_br_clr "Color [R G B] (0-1)"; tensioner_br_opc "Opacity (0.1)"; tensioner_eqpos "Equilibrium Position (m)"; tensioner_x0 "Assembly Position (m)"; tensioner_k "Stiffness Coefficient (N/m)"; tensioner_b "Damping Coefficient (N/(m/s))"; roller_upper_x "Upper Rollers (vector) (m)"; roller_lower_x "Lower Rollers (vector) (m)"; idler_x "Idler Wheel (m)"; roller_upper_y "Sprocket to Upper Rollers (m)"; plate_h "Chain Plate Height (m)"; sprk_pitch_rad "Sprocket Pitch Radius (m)"; idler_lower_roller_offset_y "Idler to Lower Roller Offset (lower edge) (m)"; popup_sense_roller "Roller"
      mask help: Models sprocket, rollers, and idler with tensioner. Components have contact geometry for integration with a segmented track model. Contact forces within the track are planar to speed up simulation. The sprocket has a 1D rotational mechanical interface to the drivetrain.
      mask TypeOptions sprk_xc: Rollers/sprk_xc
      mask TypeOptions sprk_len: Rollers/sprk_len
      mask TypeOptions sprk_rho: Rollers/sprk_rho
      mask TypeOptions sprk_clr: Rollers/sprk_clr
      mask TypeOptions sprk_opc: Rollers/sprk_opc
      mask TypeOptions sprk_contact_geo_ptcld: Rollers/sprk_contact_geo_ptcld
      mask TypeOptions sprk_contact_geo_rad: Rollers/sprk_contact_geo_rad
      mask TypeOptions sprk_contact_geo_clr: Rollers/sprk_contact_geo_clr
      mask TypeOptions sprk_contact_geo_opc: Rollers/sprk_contact_geo_opc
      mask TypeOptions idler_rad: Frame/idler_rad | Rollers/idler_rad
      mask TypeOptions idler_len: Rollers/idler_len
      mask TypeOptions idler_rho: Rollers/idler_rho
      mask TypeOptions idler_clr: Rollers/idler_clr
      mask TypeOptions idler_opc: Rollers/idler_opc
      mask TypeOptions idler_contgeo_clr: Rollers/idler_contgeo_clr
      mask TypeOptions idler_contgeo_opc: Rollers/idler_contgeo_opc
      mask TypeOptions roller_upper_rad: Rollers/roller_upper_rad
      mask TypeOptions roller_upper_len: Rollers/roller_upper_len
      mask TypeOptions roller_upper_rho: Rollers/roller_upper_rho
      mask TypeOptions roller_upper_clr: Rollers/roller_upper_clr
      mask TypeOptions roller_upper_opc: Rollers/roller_upper_opc
      mask TypeOptions roller_upper_contgeo_clr: Rollers/roller_upper_contgeo_clr
      mask TypeOptions roller_upper_contgeo_opc: Rollers/roller_upper_contgeo_opc
      mask TypeOptions roller_lower_rad: Frame/roller_lower_rad | Rollers/roller_lower_rad
      mask TypeOptions roller_lower_len: Rollers/roller_lower_len
      mask TypeOptions roller_lower_rho: Rollers/roller_lower_rho
      mask TypeOptions roller_lower_clr: Rollers/roller_lower_clr
      mask TypeOptions roller_lower_opc: Rollers/roller_lower_opc
      mask TypeOptions roller_lower_contgeo_clr: Rollers/roller_lower_contgeo_clr
      mask TypeOptions roller_lower_contgeo_opc: Rollers/roller_lower_contgeo_opc
      mask TypeOptions tensioner_cyl_len: Rollers/tensioner_cyl_len
      mask TypeOptions tensioner_cyl_rad: Rollers/tensioner_cyl_rad
      mask TypeOptions tensioner_cyl_rho: Rollers/tensioner_cyl_rho
      mask TypeOptions tensioner_cyl_clr: Rollers/tensioner_cyl_clr
      mask TypeOptions tensioner_cyl_opc: Rollers/tensioner_cyl_opc
      mask TypeOptions tensioner_pist_len: Rollers/tensioner_pist_len
      mask TypeOptions tensioner_pist_rad: Rollers/tensioner_pist_rad
      mask TypeOptions tensioner_pist_rho: Rollers/tensioner_pist_rho
      mask TypeOptions tensioner_pist_clr: Rollers/tensioner_pist_clr
      mask TypeOptions tensioner_pist_opc: Rollers/tensioner_pist_opc
      mask TypeOptions tensioner_br_length: Rollers/tensioner_br_length
      mask TypeOptions tensioner_br_width: Rollers/tensioner_br_width
      mask TypeOptions tensioner_br_height: Rollers/tensioner_br_height
      mask TypeOptions tensioner_br_thk: Rollers/tensioner_br_thk
      mask TypeOptions tensioner_br_rho: Rollers/tensioner_br_rho
      mask TypeOptions tensioner_br_clr: Rollers/tensioner_br_clr
      mask TypeOptions tensioner_br_opc: Rollers/tensioner_br_opc
      mask TypeOptions tensioner_eqpos: Rollers/tensioner_eqpos
      mask TypeOptions tensioner_x0: Rollers/tensioner_x0
      mask TypeOptions tensioner_k: Rollers/tensioner_k
      mask TypeOptions tensioner_b: Rollers/tensioner_b
      mask TypeOptions roller_upper_x: Frame/roller_upper_x
      mask TypeOptions roller_lower_x: Frame/roller_lower_x
      mask TypeOptions idler_x: Frame/idler_x
      mask TypeOptions roller_upper_y: Frame/roller_upper_y
      mask TypeOptions plate_h: Frame/plate_h
      mask TypeOptions sprk_pitch_rad: Frame/sprk_pitch_rad
      mask TypeOptions idler_lower_roller_offset_y: Frame/idler_lower_roller_offset_y
      mask TypeOptions popup_sense_roller: Rollers/popup_sense_roller
      mask DialogControl cont_sprocket Prompt: Sprocket
      mask DialogControl cont_sprocket_solid Prompt: Solid
      mask DialogControl cont_sprocket_contact_geo Prompt: Contact Geometry
      mask DialogControl cont_idler Prompt: Idler
      mask DialogControl cont_idler_solid Prompt: Solid
      mask DialogControl cont_idler_contact_geo Prompt: Contact Geometry
      mask DialogControl cont_rollers Prompt: Rollers
      mask DialogControl cont_roller_upper Prompt: Upper
      mask DialogControl cont_roller_upper_contact_geo Prompt: Contact Geometry
      mask DialogControl cont_rollers_lower Prompt: Lower
      mask DialogControl cont_rollers_lower_contact_geo Prompt: Contact Geometry
      mask DialogControl cont_tensioner Prompt: Tensioner
      mask DialogControl cont_tensioner_cyl Prompt: Cylinder
      mask DialogControl cont_tensioner_pist Prompt: Piston
      mask DialogControl cont_tensioner_brkt Prompt: Bracket
      mask DialogControl cont_tensioner_assembly Prompt: Assembly
      mask DialogControl cont_frame Prompt: Frame
      mask DialogControl cont_offset_x Prompt: Longitudinal Offsets from Sprocket
      mask DialogControl cont_offset_y Prompt: Vertical Offsets
      mask DialogControl cont_sensing Prompt: Sensing
      mask Display:
      | image('sm_excv_track_rollers_IMAGE.png');
      | disp('Pla');
